simulink model "PWMdelays"  (R2016a)
settings: Solver=VariableStepAuto  StartTime=0.0  StopTime=0.02  RelTol=1e-3
libraries: simulink x8, powerlib x1
settings Model: Creator=Alin anto  LastModifiedBy=Alin anto

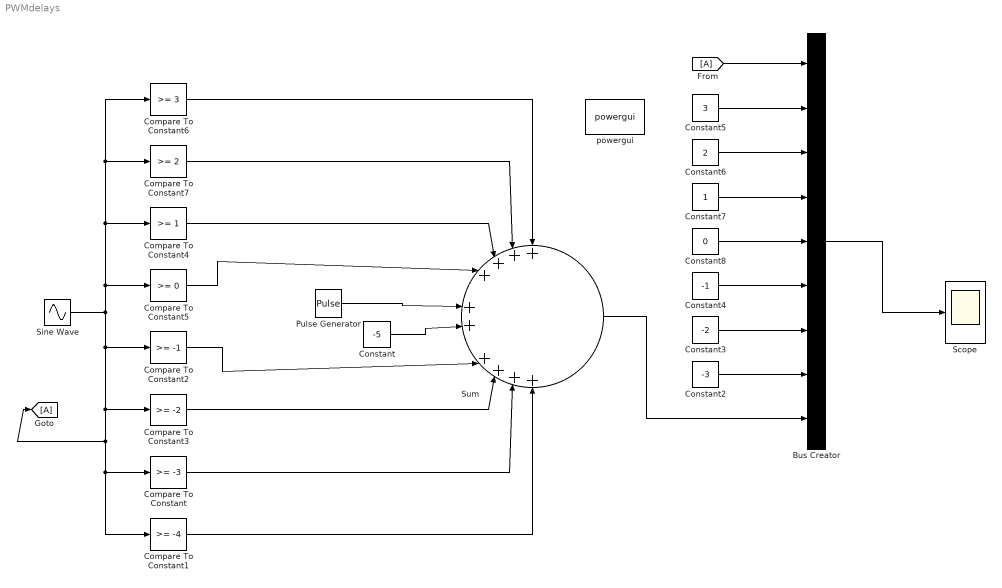
== system PWMdelays ==
  Bus Creator : BusCreator  Inputs=9
  Compare To Constant : simulink/Logic and Bit Operations/Compare To Constant  relop=>=  const=-3  OutDataTypeStr=boolean
  Compare To Constant1 : simulink/Logic and Bit Operations/Compare To Constant  relop=>=  const=-4  OutDataTypeStr=boolean
  Compare To Constant2 : simulink/Logic and Bit Operations/Compare To Constant  relop=>=  const=-1  OutDataTypeStr=boolean
  Compare To Constant3 : simulink/Logic and Bit Operations/Compare To Constant  relop=>=  const=-2  OutDataTypeStr=boolean
  Compare To Constant4 : simulink/Logic and Bit Operations/Compare To Constant  relop=>=  const=1  OutDataTypeStr=boolean
  Compare To Constant5 : simulink/Logic and Bit Operations/Compare To Constant  relop=>=  const=0  OutDataTypeStr=boolean
  Compare To Constant6 : simulink/Logic and Bit Operations/Compare To Constant  relop=>=  const=3  OutDataTypeStr=boolean
  Compare To Constant7 : simulink/Logic and Bit Operations/Compare To Constant  relop=>=  const=2  OutDataTypeStr=boolean
  Constant : Constant  Value=-5
  Constant2 : Constant  Value=-3
  Constant3 : Constant  Value=-2
  Constant4 : Constant  Value=-1
  Constant5 : Constant  Value=3
  Constant6 : Constant  Value=2
  Constant7 : Constant
  Constant8 : Constant  Value=0
  Pulse Generator : DiscretePulseGenerator  PulseType=Time based  Period=0.0001  PulseWidth=50
  Scope : Scope
  Sine Wave : Sin  Amplitude=4  Frequency=2*pi*50  SampleTime=0
  Sum : Sum  Inputs=++++|++|++++
  powergui : powerlib/powergui  Priority=1  SimulationMode=Continuous  SolverType=Tustin/Backward Euler (TBE)  SampleTime=50e-6  frequency=60  SPID=off  DisableSnubberDevices=off  DisableRonSwitches=off  DisableVfSwitches=off  SwTol=0  DisplayEquations=off  Interpol=off  ExternalGateDelay=off  methode=off  Ts=10  FunctionMessages=off  echomessages=off  HookPort=off  EnableUseOfTLC=off  x0status=blocks  frequencyindice=60  Pbase=100e6  ErrMax=1e-4  Iterations=50  UnitsV=kV  UnitsW=MW  buscounter=0  RestoreLinks=warning  ResistiveCurrentMeasurement=off  Frange=[0:2:500]  Ylog=off  Xlog=on  ShowGrid=off  save=off  variable=ZData  structure=0  ZoomFFT=off  StartTime=0.0  cycles=1  DisplayStyle=1  fundamental=60  FreqAxis=off  MaxFrequency=1000  frequencyindicesteady=1  RmsSteady=1  display=off
  wires:
  Sine Wave/1 -> [A], Compare To Constant1/1, Compare To Constant/1, Compare To Constant3/1, Compare To Constant2/1, Compare To Constant5/1, Compare To Constant4/1, Compare To Constant7/1, Compare To Constant6/1
  Pulse Generator/1 -> Sum/5
  Compare To Constant6/1 -> Sum/1
  Compare To Constant7/1 -> Sum/2
  Compare To Constant4/1 -> Sum/3
  Compare To Constant5/1 -> Sum/4
  [A] -> Bus Creator/1
  Constant5/1 -> Bus Creator/2
  Constant6/1 -> Bus Creator/3
  Constant7/1 -> Bus Creator/4
  Constant8/1 -> Bus Creator/5
  Constant4/1 -> Bus Creator/6
  Constant3/1 -> Bus Creator/7
  Constant2/1 -> Bus Creator/8
  Sum/1 -> Bus Creator/9
  Bus Creator/1 -> Scope/1
  Compare To Constant1/1 -> Sum/10
  Compare To Constant/1 -> Sum/9
  Compare To Constant3/1 -> Sum/8
  Compare To Constant2/1 -> Sum/7
  Constant/1 -> Sum/6
